simulink model "Worked_Example_5_3"  (R2024b)
settings: Solver=VariableStepAuto  StartTime=0.0  StopTime=30  RelTol=1e-3
settings Model: Creator=GH-X-ST  LastModifiedBy=GH-X-ST

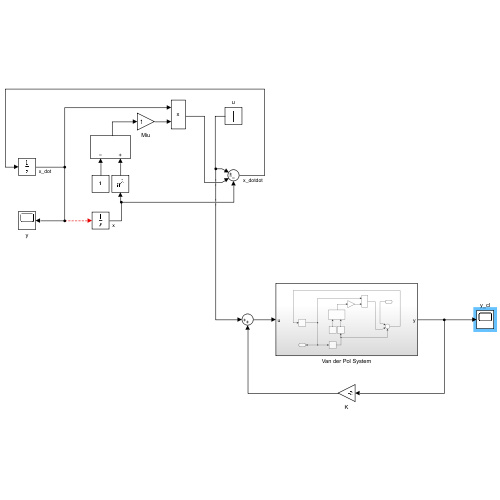
[thumbnail: Simulink's stored preview of the top-level diagram]
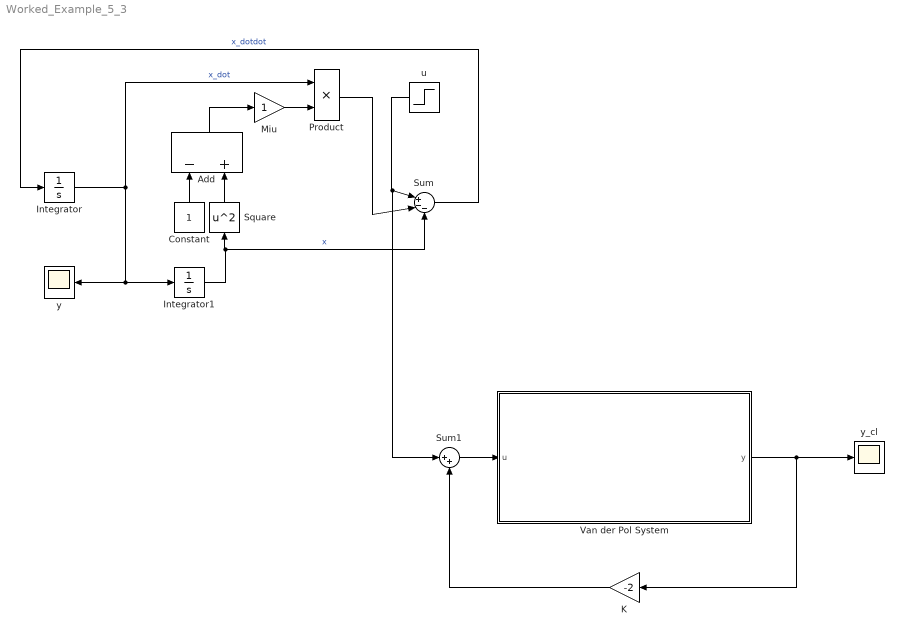
== system Worked_Example_5_3 ==
  Add : Sum  Inputs=-+
  Constant : Constant
  Integrator : Integrator  InitialCondition=0.1
  Integrator1 : Integrator  InitialCondition=0.1
  K : Gain  Gain=-2
  Miu : Gain
  Product : Product
  Square : Math  Operator=square
  Sum : Sum  Inputs=|+--
  Sum1 : Sum  Inputs=|++
  Van der Pol System : Subsystem
  u : Step  After=0  SampleTime=0
  y : Scope
  y_cl : Scope
  wires:
  u/1 -> Sum1/1, Sum/1
  Integrator/1 -> Integrator1/1, y/1, Product/1  "x_dot"
  Integrator1/1 -> Sum/3, Square/1  "x"
  Square/1 -> Add/2
  Constant/1 -> Add/1
  Add/1 -> Miu/1
  Miu/1 -> Product/2
  Product/1 -> Sum/2
  Sum/1 -> Integrator/1  "x_dotdot"
  Van der Pol System/1(y) -> K/1, y_cl/1
  K/1 -> Sum1/2
  Sum1/1 -> Van der Pol System/1(u)

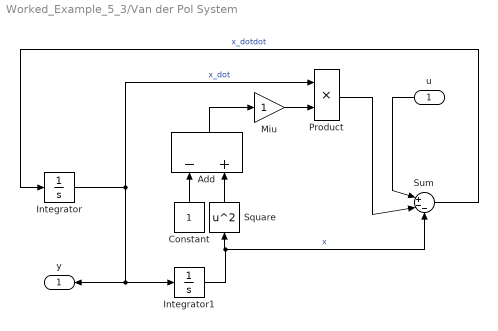
== system Worked_Example_5_3/Van der Pol System ==
  u : Inport
  Add : Sum  Inputs=-+
  Constant : Constant
  Integrator : Integrator  InitialCondition=0.1
  Integrator1 : Integrator  InitialCondition=0.1
  Miu : Gain
  Product : Product
  Square : Math  Operator=square
  Sum : Sum  Inputs=|+--
  y : Outport
  wires:
  Add/1 -> Miu/1
  Product/1 -> Sum/2
  Constant/1 -> Add/1
  u/1 -> Sum/1
  Square/1 -> Add/2
  Sum/1 -> Integrator/1  "x_dotdot"
  Integrator1/1 -> Sum/3, Square/1  "x"
  Integrator/1 -> y/1, Integrator1/1, Product/1  "x_dot"
  Miu/1 -> Product/2
